simulink model "exampleCollectorUnglazed"  (Simulink 7.6)
settings: Solver=ode45  StartTime=0.0  StopTime=24*3600  RelTol=1e-5  AbsTol=1e-5
libraries: carnot x5
settings Model: Creator=drhf  LastModifiedBy=drhf
settings CodeAppCC: CustomSymbolStrType=$N$R$M_T

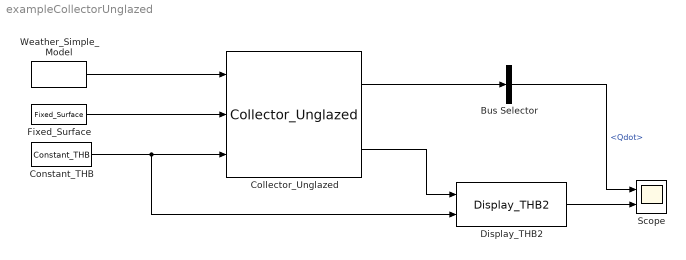
== system exampleCollectorUnglazed ==
  Bus Selector : BusSelector  OutputSignals=Qdot
  Collector_Unglazed : carnot/Source/Solar_Thermal/Collector_Unglazed  SystemSampleTime=-1  acol=2.33  len=5  fta=0.9  e_sky=0.9  uc0=10  uc1=3  uc0loss=4  uc1loss=1.5  uc0gain=6  uc1gain=1.5  uc1eta0=0.01  hi=100  c_abs=1e4  c_fl=1e2  lin=0  qua=0  tini=20  nodes=2
  Constant_THB : carnot/Source/Simple/Constant_THB  SystemSampleTime=-1  t=40  mdot=100/3600  p=1e5  mID=No Pressure Drop  fluid=water  mix=0  dia=0.02  hgt=0
  Display_THB2 : carnot/Outputs/Display_THB2  SystemSampleTime=-1  t=on  m=off  p=off  id=off  mix=off  d=off
  Fixed_Surface : carnot/Weather/Fixed_Surface  SystemSampleTime=-1  colangle=30  colazi=0  colrot=0
  Scope : Scope  NumInputPorts=2
      settings: YMin=37~-5  YMax=53~5
  Weather_Simple_Model : carnot/Weather/Weather_Simple_Model  SystemSampleTime=-1  lat=60  Ibn=900  Idg=100  tamb=5  deltaTsky=-6  rh=50  precip="10e-3/24/3600           % 10 mm in 24 h"  cloud=0.125  p=1013e2  vw=1  wdir=270
  wires:
  Weather_Simple_Model/1 -> Collector_Unglazed/1
  Fixed_Surface/1 -> Collector_Unglazed/2
  Constant_THB/1 -> Display_THB2/2, Collector_Unglazed/3
  Collector_Unglazed/2 -> Display_THB2/1
  Display_THB2/1 -> Scope/2
  Collector_Unglazed/1 -> Bus Selector/1
  Bus Selector/1 -> Scope/1  "<Qdot>"
